simulink model "untitled2"  (R2023a)
settings: Solver=VariableStepAuto  StartTime=0.0  StopTime=12  RelTol=1e-3
settings Model: Creator=User  LastModifiedBy=User

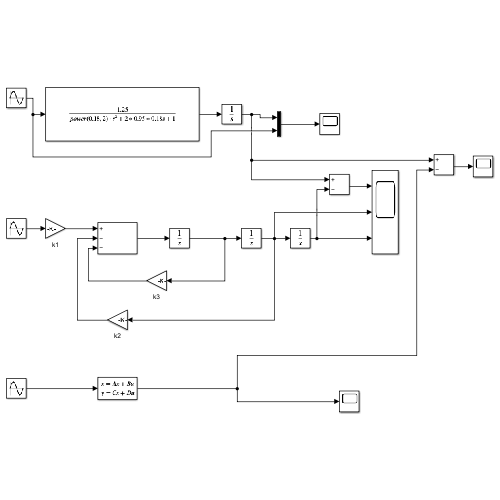
[thumbnail: Simulink's stored preview of the top-level diagram]
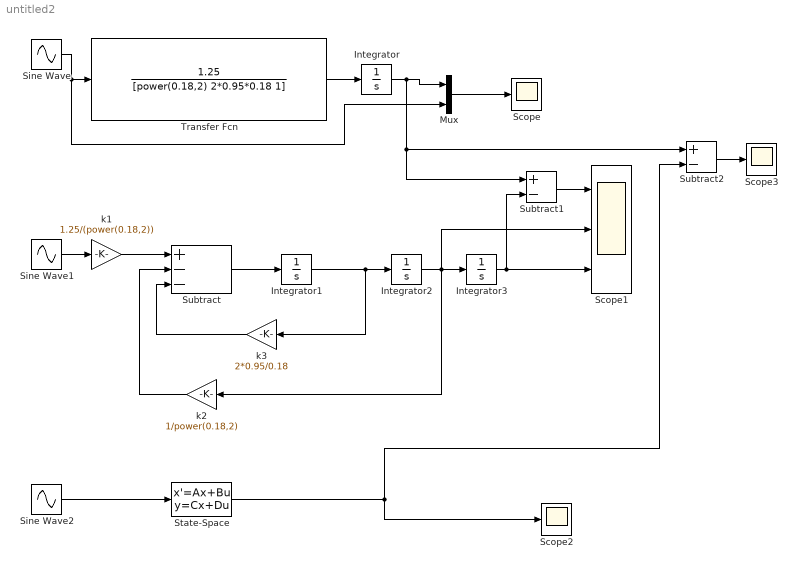
== system untitled2 ==
  Integrator{,1..3} (4 alike) : Integrator
  Mux : Mux  Inputs=2
  Scope : Scope
  Scope1 : Scope  NumInputPorts=3
  Scope2 : Scope
  Scope3 : Scope
  Sine Wave : Sin  SampleTime=0
  Sine Wave1 : Sin  SampleTime=0
  Sine Wave2 : Sin  SampleTime=0
  State-Space : StateSpace  A=[0 1 0; 0 0 1; 0 -(1/power(0.18,2)) -(2*0.95/0.18)]  B=[0; 0; 1]  C=[(1.25/power(0.18,2)) 0 0]  D=0  InitialCondition=0
  Subtract : Sum  Inputs=+--
  Subtract1 : Sum  Inputs=+-
  Subtract2 : Sum  Inputs=+-
  Transfer Fcn : TransferFcn  Numerator=[1.25]  Denominator=[power(0.18,2) 2*0.95*0.18 1]
  k1 : Gain  Gain=1.25/(power(0.18,2))
  k2 : Gain  Gain=1/power(0.18,2)
  k3 : Gain  Gain=2*0.95/0.18
  wires:
  Transfer Fcn/1 -> Integrator/1
  Integrator/1 -> Subtract2/1, Subtract1/1, Mux/1
  Sine Wave/1 -> Mux/2, Transfer Fcn/1
  Mux/1 -> Scope/1
  Sine Wave1/1 -> k1/1
  k1/1 -> Subtract/1
  Subtract/1 -> Integrator1/1
  Integrator1/1 -> Integrator2/1, k3/1
  Integrator2/1 -> Scope1/2, Integrator3/1, k2/1
  k3/1 -> Subtract/3
  Integrator3/1 -> Subtract1/2, Scope1/3
  k2/1 -> Subtract/2
  Subtract1/1 -> Scope1/1
  Sine Wave2/1 -> State-Space/1
  State-Space/1 -> Subtract2/2, Scope2/1
  Subtract2/1 -> Scope3/1
